simulink model "dsm_example"  (R2014b)
settings: Solver=FixedStepDiscrete  StartTime=0.0  StopTime=5  FixedStep=0.1  RelTol=1e-3
PreLoadFcn:
  | %   Copyright 2014 The MathWorks, Inc.
  | 
  | dsm = Simulink.Signal;
  | dsm.DataType = 'double';
  | dsm.SamplingMode = 'Sample based';
  | dsm.InitialValue = '5.0';
  | dsm.StorageClass = 'ExportedGlobal';
  | dsm.Complexity = 'real';
  | dsm.Description = 'dsm_description';
settings Model: Creator=The MathWorks Inc.  LastModifiedBy=vselvam
settings DataIOCC: SignalLoggingSaveFormat=ModelDataLogs
settings OptimizationCC: ExpressionDepthLimit=2147483647  InitFltsAndDblsToZero=on  EfficientMapNaN2IntZero=off  OptimizeModelRefInitCode=on  LifeSpan=1
settings DebuggingCC: ReadBeforeWriteMsg=DisableAll  WriteAfterWriteMsg=DisableAll  WriteAfterReadMsg=DisableAll  UnderspecifiedInitializationDetection=Classic  MergeDetectMultiDrivingBlocksExec=none  MultiTaskDSMMsg=none  FcnCallInpInsideContextMsg=UseLocalSettings  UniqueDataStoreMsg=error  StateNameClashWarn=warning
settings SFSimCC: SimParseCustomCode=off
settings RTWCC: SystemTargetFile=ert.tlc  GenCodeOnly=on  TemplateMakefile=ert_default_tmf  Description=Embedded Coder  RetainRTWFile=on  ProcessScript=ert_make_rtw_hook
settings CodeAppCC: IgnoreCustomStorageClasses=off
settings ERTTargetCC: GenerateSampleERTMain=on  SupportContinuousTime=on  ERTCustomFileTemplate=example_file_process.tlc
settings ConfigComp: Description=Design Verifier Custom Configuration Component  DVMaxProcessTime=600  DVDisplayUnsatisfiableObjectives=on  DVAutomaticStubbing=off  DVParameters=on  DVModelCoverageObjectives=MCDC  DVMaxTestCaseSteps=500  DVTestSuiteOptimization=CombinedObjectives  DVDetectActiveLogic=on  DVSaveHarnessModel=on  DVSaveReport=on  PLC_OutputDir=notb  PLC_TargetIDE=omron  PLC_ExternalDefinedNames=dsm

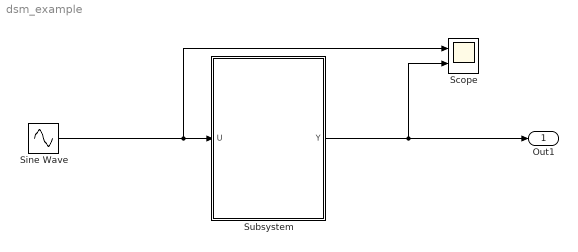
== system dsm_example ==
  Scope : Scope  NumInputPorts=2
      settings: YMin=-5~-5  YMax=5~5
  Sine Wave : Sin  SampleTime=0
  Subsystem : Subsystem  TreatAsAtomicUnit=on
  Out1 : Outport
  wires:
  Subsystem/1(Y) -> Scope/2, Out1/1
  Sine Wave/1 -> Subsystem/1(U), Scope/1

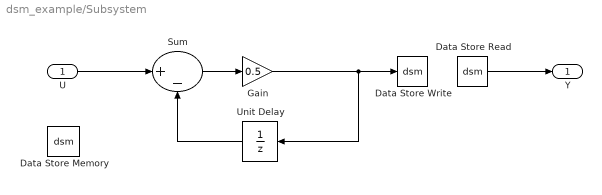
== system dsm_example/Subsystem ==
  U : Inport  OutDataTypeStr=double
  Data Store Memory : DataStoreMemory  DataStoreName=dsm  ReadBeforeWriteMsg=warning  WriteAfterWriteMsg=warning  WriteAfterReadMsg=warning  InitialValue=[]  StateMustResolveToSignalObject=on
  Data Store Read : DataStoreRead  DataStoreName=dsm
  Data Store Write : DataStoreWrite  DataStoreName=dsm
  Gain : Gain  Gain=0.5
  Sum : Sum  Inputs=|+-
  Unit Delay : UnitDelay  SampleTime=-1
  Y : Outport
  wires:
  Sum/1 -> Gain/1
  U/1 -> Sum/1
  Unit Delay/1 -> Sum/2
  Gain/1 -> Data Store Write/1, Unit Delay/1
  Data Store Read/1 -> Y/1
